simulink model "Wischer_Box17b"  (R2017b)
settings: Solver=FixedStepAuto  StartTime=0.0  StopTime=10.0  RelTol=1e-3
PreLoadFcn:
  | waijung.modelPreload; % Required for working with Waijung Blockset. Do not remove.
undefined symbols (not defined in the file): HSEOSC, Link, LQFP176, ST, STM32F417IG
libraries: simulink x12, canmsglib x6, stm32f4_canbus_lib x3, hdlsllib x2, stm32f4_io_lib x2, stm32f4_adc_lib x1, stm32f4_device_config_lib x1
CloseFcn:
  | waijung.modelClose; % Required for working with Waijung Blockset. Do not remove.
settings Model: Creator=id605605  LastModifiedBy=MichaelRogalski
settings DataIOCC: ReturnWorkspaceOutputs=on
settings OptimizationCC: DefaultParameterBehavior=Inlined  EnhancedBackFolding=on  PassReuseOutputArgsAs=Individual arguments  ZeroExternalMemoryAtStartup=off  ZeroInternalMemoryAtStartup=off  OptimizeBlockOrder=speed  DifferentSizesBufferReuse=on
settings DebuggingCC: ParameterTunabilityLossMsg=error
settings HardwareCC: ProdBitPerPointer=32  ProdBitPerSizeT=32  ProdBitPerPtrDiffT=32  ProdLargestAtomicFloat=None  ProdIntDivRoundTo=Undefined  ProdWordSize=32  ProdHWDeviceType=ARM Compatible->Cortex - M4  TargetEndianess=LittleEndian  TargetHWDeviceType=ARM Compatible->Cortex - M4
settings SFSimCC: SimUseLocalCustomCode=on  MATLABDynamicMemAlloc=off
settings RTWCC: Description=STM32F4 Target  SystemTargetFile=stm32f4.tlc  GenerateMakefile=off  TemplateMakefile=ert_default_tmf  GenerateReport=on  RTWUseLocalCustomCode=on  IncludeHyperlinkInReport=on  LaunchReport=on  GenerateTraceInfo=on  GenerateTraceReport=on  GenerateTraceReportSl=on  GenerateTraceReportSf=on  GenerateTraceReportEml=on
settings CodeAppCC: ForceParamTrailComments=on  IgnoreCustomStorageClasses=off  OperatorAnnotations=on  SimulinkDataObjDesc=on  SFDataObjDesc=on  InsertBlockDesc=on
settings STFCustomTargetCC: TargetLangStandard=C99 (ISO)  MultiwordLength=256  ModelReferenceCompliant=off  CombineOutputUpdateFcns=on  ERTCustomFileBanners=on  SupportContinuousTime=off  SupportNonInlinedSFcns=off  RemoveResetFunc=on  MATLABClassNameForMDSCustomization=Simulink.SoftwareTarget.ERTCustomization  GRTInterface=off  SystemTargetFile=stm32f4.tlc
settings ERTTargetCC: TargetLangStandard=C99 (ISO)  ModelReferenceCompliant=off  ParMdlRefBuildCompliant=off  CompOptLevelCompliant=off  ConcurrentExecutionCompliant=off  ModelStepFunctionPrototypeControlCompliant=off  CPPClassGenCompliant=off  UseToolchainInfoCompliant=off  InlinedParameterPlacement=NonHierarchical  ERTSrcFileBannerTemplate=stm32f4_code_template.cgt  ERTHdrFileBannerTemplate=stm32f4_code_template.cgt  ERTDataSrcFileTemplate=stm32f4_code_template.cgt  ERTDataHdrFileTemplate=stm32f4_code_template.cgt  ERTCustomFileTemplate=stm32f4_file_process.tlc

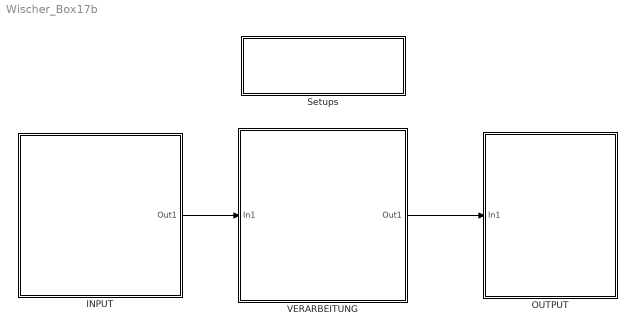
== system Wischer_Box17b ==
  INPUT : Subsystem
  OUTPUT : Subsystem
  Setups : Subsystem
  VERARBEITUNG : Subsystem
  wires:
  VERARBEITUNG/1(Out1) -> OUTPUT/1(In1)
  INPUT/1(Out1) -> VERARBEITUNG/1(In1)

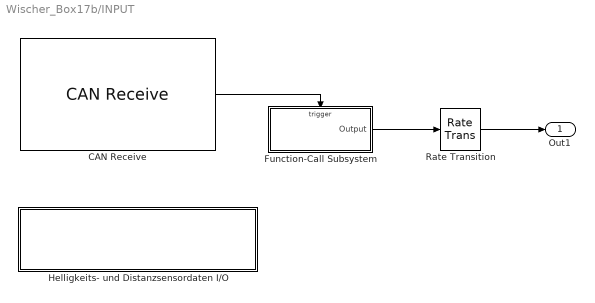
== system Wischer_Box17b/INPUT ==
  CAN Receive : stm32f4_canbus_lib/CAN Receive  conf=Rx  canmodule=1  idtype=Standard  filtertype=Mask  id=0  idmask=0  enableisr=on  usedlc=off  datatype=single  data0type=uint32  data1type=uint32  data2type=Not used  data3type=Not used  data4type=Not used  data5type=Not used  data6type=Not used  data7type=Not used  buffersize=8  sampletime=-1  sampletimestr=-1  blockid=INPUTCANReceive  inputarray=[]  inputlabelarray={}  outputarray=[7]  outputlabelarray={'Call ISR' }  compat=0  confstr=[]
      settings: SourceProductName=Waijung Blockset
  Function-Call Subsystem : Subsystem  TreatAsAtomicUnit=on
  Helligkeits- und Distanzsensordaten I/O : Subsystem
  Rate Transition : RateTransition
  Out1 : Outport  VectorParamsAs1DForOutWhenUnconnected=off
  wires:
  CAN Receive/1 -> Function-Call Subsystem/Trigger
  Function-Call Subsystem/1(Output) -> Rate Transition/1
  Rate Transition/1 -> Out1/1

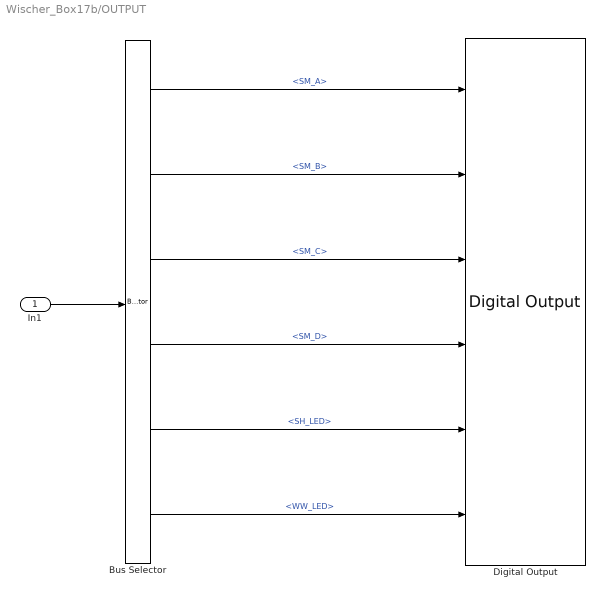
== system Wischer_Box17b/OUTPUT ==
  In1 : Inport
  Bus Selector : BusSelector  OutputSignals=SM_A,SM_B,SM_C,SM_D,SH_LED,WW_LED
  Digital Output : stm32f4_io_lib/Digital Output  use_bitband=on  port=C  speed=100  porttype=Push Pull  porttypestr=PP  use_pin0=on  use_pin1=on  use_pin2=on  use_pin3=on  use_pin4=on  use_pin5=on  use_pin6=off  use_pin7=off  use_pin8=off  use_pin9=off  use_pin10=off  use_pin11=off  use_pin12=off  use_pin13=off  use_pin14=off  use_pin15=off  pinstr=GPIO_Pin_0 | GPIO_Pin_1 | GPIO_Pin_2 | GPIO_Pin_3 | GPIO_Pin_4 | GPIO_Pin_5  usedpinarray="[1  1  1  1  1  1  0  0  0  0  0  0  0  0  0  0]"  bitbandingstr=|  sampletime=-1  sampletimestr=-1  blockid=OUTPUTDigitalOutput  enablecustomportlabel=off  globalinit=off  cinputportlabel=In1, In2  coutputportlabel=0
      | #define OUTPUTDigitalOutput_C0 Peripheral_BB(GPIOC->ODR, 0)  /* Output pin */
      | #define OUTPUTDigitalOutput_C1 Peripheral_BB(GPIOC->ODR, 1)  /* Output pin */
      | #define OUTPUTDigitalOutput_C2 Peripheral_BB(GPIOC->ODR, 2)  /* Output pin */
      | #define OUTPUTDigitalOutput_C3 Peripheral_BB(GPIOC->ODR, 3)  /* Output pin */
      | #define OUTPUTDigitalOutput_C4 Peripheral_BB(GPIOC->ODR, 4)  /* Output pin */
      | #define OUTPUTDigitalOutput_C5 Peripheral_BB(GPIOC->ODR, 5)  /* Output pin */
      settings: SourceProductName=Waijung Blockset
  wires:
  In1/1 -> Bus Selector/1
  Bus Selector/1 -> Digital Output/1  "<SM_A>"
  Bus Selector/2 -> Digital Output/2  "<SM_B>"
  Bus Selector/3 -> Digital Output/3  "<SM_C>"
  Bus Selector/4 -> Digital Output/4  "<SM_D>"
  Bus Selector/6 -> Digital Output/6  "<WW_LED>"
  Bus Selector/5 -> Digital Output/5  "<SH_LED>"

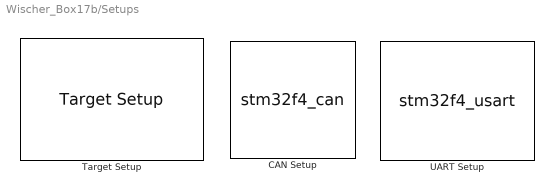
== system Wischer_Box17b/Setups ==
  CAN Setup : S-Function  FunctionName=stm32f4_can  Parameters=conf,canmodule,0,inputarray,outputarray,'','',confstr,sampletime,sampletimestr,blockid  SFunctionDeploymentMode=off  EnableBusSupport=off  mask(stm32f4_can){conf=Setup, canmodule=1, advance=off, bitrate_select=500000, sjw=1tq, bs1=14tq, bs2=6tq, timingconf=Prescaler, brp=4, bitrate=500000, tq=9.5238e-08, autoretransmission=Disable, remaptxpin=A12, remaprxpin=A11, sampletime=-1, sampletimestr=-1, blockid=SetupsCANSetup, inputarray=[], inputlabelarray={}, outputarray=[], outputlabelarray={}, compat=0, confstr=[], presc=4, txportstr=A, txpinstr=12, rxportstr=A, rxpinstr=11, lastmodule=1}
      mask prompts: conf "Configuration"; canmodule "CAN Module"; advance "Advance configuration"; bitrate_select "Baud rate (bps)"; sjw "Resync Jump Width (SJW)"; bs1 "Bit segment 1 (BS1) + PROP_SEG"; bs2 "Bit segment 2 (BS2)"; timingconf "Adjust"; brp "Baud rate prescaler (BRP)"; bitrate "Baud rate (bps)"; tq "Time Quantum (Second), tq"; autoretransmission "Auto Re-transmission"; remaptxpin "CAN Tx pin"; remaprxpin "CAN Rx pin"; sampletime "Sample time (sec)"; sampletimestr "Compiled sample time (sec) in string"; inputarray "Input port"; inputlabelarray "Input port label"; outputarray "Output port"; outputlabelarray "Output port label"; compat "Compatibility (Reserved for future use)"; confstr "Configuration String"; presc "Prescale"; txportstr "Tx port string"; txpinstr "Tx pin string"; rxportstr "Rx port string"; rxpinstr "Rx pin string"; lastmodule "Last module selected"
      mask help:
      | This block setups CAN Module.
      |
      | Auto Re-transmission,
      |  - Enable: The CAN hardware will automatically retransmit the message until it has been
      | successfully transmitted according to the CAN standard.
      |  - Disable: A message will be transmitted only once, independently of the transmission result
      | (successful, error or arbitration lost).
      mask init:
      | stm32f4_can_callback('init');
      mask Help: web(fullfile(waijungdocroot,'stm32f4_can_setup.htm'), '-browser')
      mask TypeOptions conf: Setup
      mask TypeOptions canmodule: 1 | 2
      mask Callback canmodule: stm32f4_can_callback('canmodule');
      mask Callback advance: stm32f4_can_callback('advance');
      mask TypeOptions bitrate_select: 125000 | 250000 | 500000 | 1000000
      mask Callback bitrate_select: stm32f4_can_callback('bitrate_select');
      mask TypeOptions sjw: 1tq | 2tq | 3tq | 4tq
      mask TypeOptions bs1: 1tq | 2tq | 3tq | 4tq | 5tq | 6tq | 7tq | 8tq | 9tq | 10tq | 11tq | 12tq | 13tq | 14tq | 15tq | 16tq
      mask Callback bs1: stm32f4_can_callback('timingconf');
      mask TypeOptions bs2: 1tq | 2tq | 3tq | 4tq | 5tq | 6tq | 7tq | 8tq
      mask Callback bs2: stm32f4_can_callback('timingconf');
      mask TypeOptions timingconf: Prescaler | Baudrate
      mask Callback timingconf: stm32f4_can_callback('timingconf');
      mask Callback brp: stm32f4_can_callback('timingconf');
      mask Callback bitrate: stm32f4_can_callback('timingconf');
      mask TypeOptions autoretransmission: Enable | Disable
      mask TypeOptions remaptxpin: Not used | A12 | B9 | D1 | H13
      mask Callback remaptxpin: stm32f4_can_callback('remaptxpin');
      mask TypeOptions remaprxpin: Not used | A11 | B8 | D0 | I9
      mask Callback remaprxpin: stm32f4_can_callback('remaprxpin');
      mask Callback sampletime: stm32f4_can_callback('sampletime');
      mask Callback sampletimestr: stm32f4_can_callback('sampletimestr');
      mask Callback blockid: stm32f4_can_callback('blockid');
      mask Display: text(0.5, 0.5, 'CAN1_Setup\nSpeed (bps): 500000\nTx/Rx pin: A12/A11','ver','middle','hor','center');
  Target Setup : stm32f4_device_config_lib/Target Setup  Priority=100  compiler=GNU ARM  previous_compiler=GNU ARM  mcu=STM32F417IG (LQFP176)  mcustr=STM32F417IG  clockconfig=HSEOSC-8MHz  system_stm32f4xx_c_path=D:\Downloads\waijung17_03a\targets\stm32f4_target\stm32f4\utils\system_stm32f4xx_default\STM32F40_41xxx\hseosc8mhz  showmemoryconfiguration=off  stacksize=0x2000  heapsize=0x2000  enableautocompiledownload=on  fullchiperase=off  programmerinterface=ST-Link  editctrlstr=on  compilercontrolstr=$(patsubst %, -I%, .) -mcpu=cortex-m4 -mthumb -mthumb-interwork -mfloat-abi=hard -mfpu=fpv4-sp-d16 -ffast-math -Wall -Wextra -Ofast  assemblercontrolstr=$(patsubst %, -I%, .) -mcpu=cortex-m4 -mthumb -mthumb-interwork -mfloat-abi=hard -mfpu=fpv4-sp-d16 -ffast-math -Wall -Wextra -Ofast -Wa,-amhls=$(<:.s=.lst) -D__STACK_SIZE=$(STACK_SIZE) -D__HEAP_SIZE=$(HEAP_SIZE)  linkercontrolstr=-T$(LD_SCRIPT) -g -Wl,-Map=$(MAP),--cref,--no-warn-mismatch -mcpu=cortex-m4 -mthumb -mthumb-interwork -mfloat-abi=hard -mfpu=fpv4-sp-d16 -specs=nosys.specs  runafterdownload=on  execprofile=None  profileruart=3  profilerbaud=500000  profilertxpin=D8  profilerinitstr=0.01,168000000,1680000,500000,0  manualsetsampletime=off  sampletime=0.01  blockid=SetupsTargetSetup  systickreloadvalue=1680000  hseval=8000000  lastprofileruart=3  hclk=168000000  flashorigin=0x8000000  flashlength=1024k  ramorigin=0x20000000  ramlength=128k  useextram=off
      settings: SourceProductName=Waijung Blockset
  UART Setup : S-Function  Priority=1  FunctionName=stm32f4_usart  Parameters=configuration,uartmodule,transfer,baudrate,inputtype,outputtype,confstr,binheaderarray,binterminatorarray,asciiheader,asciiterminator,bindatalength,packetmode,varname,sampletime,sampletimestr,blockid  SFunctionDeploymentMode=off  EnableBusSupport=off  mask(stm32f4_usart){configuration=Setup, uartmodule=2, baudrate=115200, databits=8, parity=No, stopbit=1, remaptxpin=A2, remaprxpin=A3, flowcontrol=None, remapctspin=Not used, remaprtspin=Not used, advanceoptions=off, rxbuffersize=512, txbuffersize=512, transfer=Blocking, packetmode=Ascii, binheader='7E 7E', binterminator='03 03', porttype_double=1, porttype_single=0, porttype_int8=1, porttype_uint8=0, porttype_int16=0, porttype_uint16=0, porttype_int32=0, porttype_uint32=0, asciiformat='%d,%f', rx_asciiterminator=CRLF (0x0D 0x0A - "\r\n"), tx_asciiterminator=CR (0x0D - "\r"), storagename=<empty>, varname=, inputtype=[0], outputtype=[0], binheaderarray=[0], binterminatorarray=[0], bindatalength=0, asciiheader='', asciiterminator=[0], sampletime=-1, sampletimestr=-1, blockid=SetupsUARTSetup, confstr=[ "dummy", "1", "A", "2", "1", "A", "3", "0", "*", "*", "0", "*", "*", "1", "4", "6", "1", "4", "5", "512", "512", "1", "2", "115200", "8", "No", "1", "None", "USART2"], lastmodule=2}
      mask prompts: uartmodule "UART Module"; baudrate "Baud rate (bps)"; databits "Data bits"; stopbit "Stop bit"; remaptxpin "Tx Pin"; remaprxpin "Rx Pin"; flowcontrol "Hardware flow control"; remapctspin "HW Flow control, CTS Pin"; remaprtspin "HW Flow control, RTS Pin"; advanceoptions "Advance options"; rxbuffersize "Rx buffer size (bytes)"; txbuffersize "Tx buffer size (bytes)"; packetmode "Packet mode"; binheader "Binary header (example: '7E 7E')"; binterminator "Binary terminator (example: '03 03')"; porttype_double "Number of data port, type DOUBLE"; porttype_single "Number of data port, type SINGLE"; porttype_int8 "Number of data port, type INT8"; porttype_uint8 "Number of data port, type UINT8"; porttype_int16 "Number of data port, type INT16"; porttype_uint16 "Number of data port, type UINT16"; porttype_int32 "Number of data port, type INT32"; porttype_uint32 "Number of data port, type UINT32"; asciiformat "Ascii format"; rx_asciiterminator "End of packet"; tx_asciiterminator "End of packet"; storagename "Buffer"; varname "Var name"; inputtype "Input data type"; outputtype "Output data type"; binheaderarray "Binary header"; binterminatorarray "Binary terminator"; bindatalength "Binary data length"; asciiheader "Ascii header (printf format)"; asciiterminator "Ascii terminator"; sampletime "Sample time (sec)"; sampletimestr "Compiled sample time (sec) in string"; confstr "Configuration string"; lastmodule "Last module selected"
      mask help:
      | Default STM32F4DISCOVERY + aMG F4 Connect 2 + aMG USB Converter N2 settings use
      |
      | USART3, Tx D8, Rx D9 and USB Serial Converter A.
      mask init:
      | stm32f4_usart_callback('init');
      mask Help: web(fullfile(waijungdocroot,'stm32f4_usart_setup.htm'), '-browser')
      mask TypeOptions configuration: Setup | Tx | Rx
      mask Callback configuration: stm32f4_usart_callback('configuration');
      mask TypeOptions uartmodule: 1 | 2 | 3 | 4 | 5 | 6
      mask Callback uartmodule: stm32f4_usart_callback('uartmodule');
      mask Callback baudrate: stm32f4_usart_callback('baudrate');
      mask TypeOptions databits: 8
      mask TypeOptions parity: No | Odd | Even
      mask TypeOptions stopbit: 0.5 | 1 | 1.5 | 2
      mask TypeOptions remaptxpin: Not used | A2 | D5
      mask TypeOptions remaprxpin: Not used | A3 | D6
      mask TypeOptions flowcontrol: None | RTS | CTS | RTS/CTS
      mask Callback flowcontrol: stm32f4_usart_callback('flowcontrol');
      mask TypeOptions remapctspin: Not used | A0 | D3
      mask TypeOptions remaprtspin: Not used | A1 | D4
      mask Callback advanceoptions: stm32f4_usart_callback('advanceoptions');
      mask TypeOptions rxbuffersize: 16 | 32 | 64 | 128 | 256 | 512 | 1024 | 2048
      mask TypeOptions txbuffersize: 16 | 32 | 64 | 128 | 256 | 512 | 1024 | 2048
      mask TypeOptions transfer: Blocking | Non-Blocking
      mask Callback transfer: stm32f4_usart_callback('transfer');
      mask TypeOptions packetmode: Ascii | Binary | String Buffer
      mask Callback packetmode: stm32f4_usart_callback('packetmode');
      mask Callback binheader: stm32f4_usart_callback('binheader');
      mask Callback binterminator: stm32f4_usart_callback('binterminator');
      mask Callback porttype_double: stm32f4_usart_callback('porttype');
      mask Callback porttype_single: stm32f4_usart_callback('porttype');
      mask Callback porttype_int8: stm32f4_usart_callback('porttype');
      mask Callback porttype_uint8: stm32f4_usart_callback('porttype');
      mask Callback porttype_int16: stm32f4_usart_callback('porttype');
      mask Callback porttype_uint16: stm32f4_usart_callback('porttype');
      mask Callback porttype_int32: stm32f4_usart_callback('porttype');
      mask Callback porttype_uint32: stm32f4_usart_callback('porttype');
      mask Callback asciiformat: stm32f4_usart_callback('asciiformat');
      mask TypeOptions rx_asciiterminator: CR (0x0D - "\r") | LF (0x0A - "\n") | CRLF (0x0D 0x0A - "\r\n")
      mask Callback rx_asciiterminator: stm32f4_usart_callback('rx_asciiterminator');
      mask TypeOptions tx_asciiterminator: CR (0x0D - "\r") | LF (0x0A - "\n") | CRLF (0x0D 0x0A - "\r\n") | None
      mask Callback tx_asciiterminator: stm32f4_usart_callback('tx_asciiterminator');
      mask TypeOptions storagename: <empty>
      mask Callback storagename: stm32f4_usart_callback('storagename');
      mask Callback varname: stm32f4_usart_callback('varname');
      mask Callback sampletime: stm32f4_usart_callback('sampletime');
      mask Callback sampletimestr: stm32f4_usart_callback('sampletimestr');
      mask Callback blockid: stm32f4_usart_callback('blockid');
      mask Display: text(0.5, 0.5, 'Module: USART2_Setup\nBaud (Bps): 115200\nDMA Buffer: 512/512\nTx/Rx Pin: A2/A3','ver','middle','hor','center');

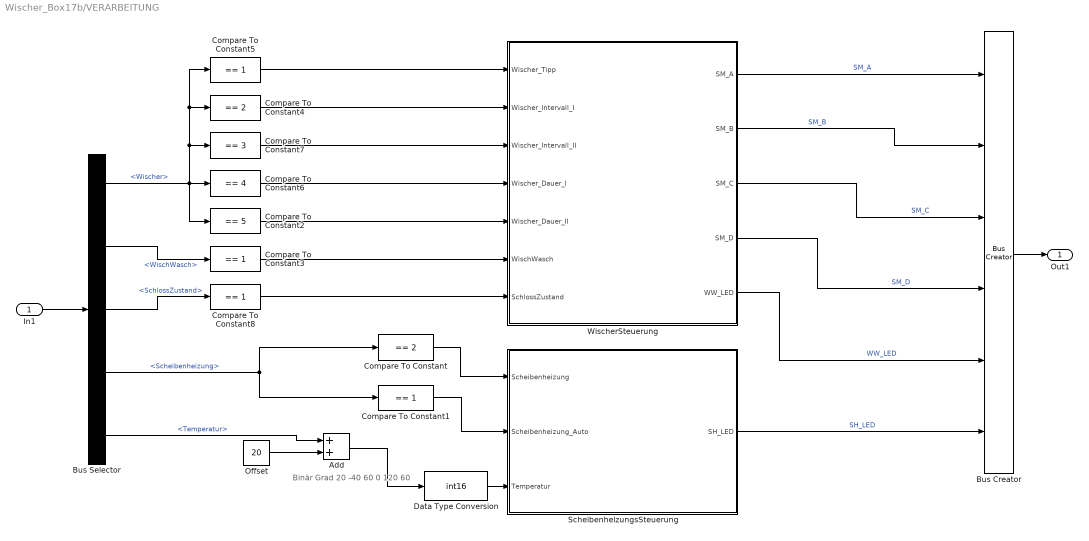
== system Wischer_Box17b/VERARBEITUNG ==
  note: Binär   Grad
      | 20		-40
      | 60		0
      | 120		60
  In1 : Inport
  Add : Sum
  Bus Creator : BusCreator  Inputs=6
  Bus Selector : BusSelector  OutputSignals=Wischer,WischWasch,SchlossZustand,Scheibenheizung,Temperatur
  Compare To Constant : simulink/Logic and Bit Operations/Compare To Constant  relop===  const=2  OutDataTypeStr=boolean
  Compare To Constant{1,3,5,8} (4 alike) : simulink/Logic and Bit Operations/Compare To Constant  relop===  const=1  OutDataTypeStr=boolean
  Compare To Constant2 : simulink/Logic and Bit Operations/Compare To Constant  relop===  const=5  OutDataTypeStr=boolean
  Compare To Constant4 : simulink/Logic and Bit Operations/Compare To Constant  relop===  const=2  OutDataTypeStr=boolean
  Compare To Constant6 : simulink/Logic and Bit Operations/Compare To Constant  relop===  const=4  OutDataTypeStr=boolean
  Compare To Constant7 : simulink/Logic and Bit Operations/Compare To Constant  relop===  const=3  OutDataTypeStr=boolean
  Data Type Conversion : DataTypeConversion  OutDataTypeStr=int16
  Offset : Constant  Value=20
  ScheibenheizungsSteuerung : Stateflow chart  TreatAsAtomicUnit=on
  WischerSteuerung : Stateflow chart  TreatAsAtomicUnit=on
  Out1 : Outport  VectorParamsAs1DForOutWhenUnconnected=off
  wires:
  Bus Creator/1 -> Out1/1
  In1/1 -> Bus Selector/1
  WischerSteuerung/1(SM_A) -> Bus Creator/1  "SM_A"
  WischerSteuerung/2(SM_B) -> Bus Creator/2  "SM_B"
  WischerSteuerung/3(SM_C) -> Bus Creator/3  "SM_C"
  WischerSteuerung/4(SM_D) -> Bus Creator/4  "SM_D"
  WischerSteuerung/5(WW_LED) -> Bus Creator/5  "WW_LED"
  ScheibenheizungsSteuerung/1(SH_LED) -> Bus Creator/6  "SH_LED"
  Bus Selector/3 -> Compare To Constant8/1  "<SchlossZustand>"
  Bus Selector/4 -> Compare To Constant/1, Compare To Constant1/1  "<Scheibenheizung>"
  Compare To Constant/1 -> ScheibenheizungsSteuerung/1(Scheibenheizung)
  Compare To Constant1/1 -> ScheibenheizungsSteuerung/2(Scheibenheizung_Auto)
  Compare To Constant7/1 -> WischerSteuerung/3(Wischer_Intervall_II)
  Compare To Constant4/1 -> WischerSteuerung/2(Wischer_Intervall_I)
  Bus Selector/1 -> Compare To Constant2/1, Compare To Constant7/1, Compare To Constant4/1, Compare To Constant5/1, Compare To Constant6/1  "<Wischer>"
  Compare To Constant6/1 -> WischerSteuerung/4(Wischer_Dauer_I)
  Compare To Constant2/1 -> WischerSteuerung/5(Wischer_Dauer_II)
  Compare To Constant5/1 -> WischerSteuerung/1(Wischer_Tipp)
  Bus Selector/2 -> Compare To Constant3/1  "<WischWasch>"
  Compare To Constant3/1 -> WischerSteuerung/6(WischWasch)
  Compare To Constant8/1 -> WischerSteuerung/7(SchlossZustand)
  Offset/1 -> Add/2
  Bus Selector/5 -> Add/1  "<Temperatur>"
  Add/1 -> Data Type Conversion/1
  Data Type Conversion/1 -> ScheibenheizungsSteuerung/3(Temperatur)

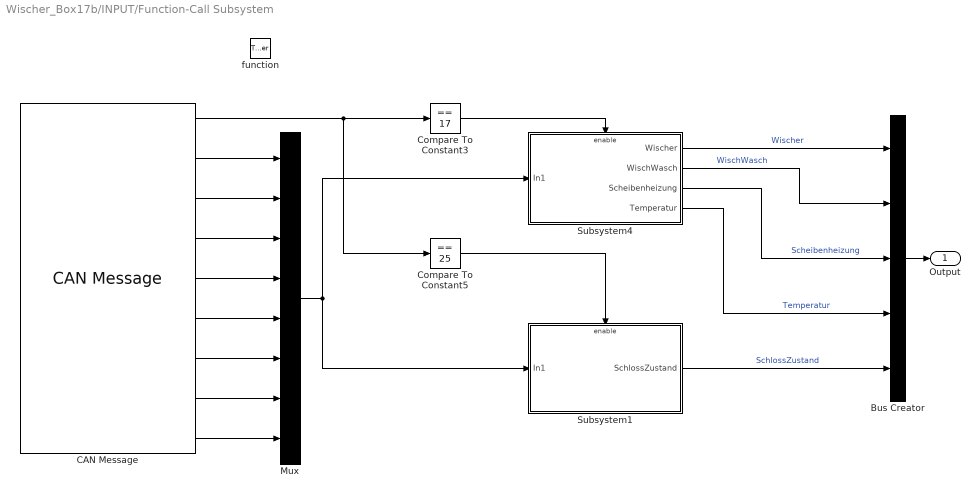
== system Wischer_Box17b/INPUT/Function-Call Subsystem ==
  function : TriggerPort  TriggerType=function-call  VariantControl=Variant
  Bus Creator : BusCreator  Inputs=5
  CAN Message : stm32f4_canbus_lib/CAN Message  conf=Msg  canmodule=1  usedlc=off  datatype=double  data0type=uint8  data1type=uint8  data2type=uint8  data3type=uint8  data4type=uint8  data5type=uint8  data6type=uint8  data7type=uint8  sampletime=-1  sampletimestr=-1  blockid=INPUTFunctionCallSubsystemCANMessage  inputarray=[]  inputlabelarray={}  outputarray=[ 7, 3, 3, 3, 3, 3, 3, 3, 3]  outputlabelarray={'ID', 'D0 (uint8)', 'D1 (uint8)', 'D2 (uint8)', 'D3 (uint8)', 'D4 (uint8)', 'D5 (uint8)', 'D6 (uint8)', 'D7 (uint8)' }  compat=0  confstr=[]
      settings: SourceProductName=Waijung Blockset
  Compare To Constant3 : simulink/Logic and Bit Operations/Compare To Constant  relop===  const=17  OutDataTypeStr=boolean
  Compare To Constant5 : simulink/Logic and Bit Operations/Compare To Constant  relop===  const=25  OutDataTypeStr=boolean
  Mux : Mux  Inputs=8
  Subsystem1 : Subsystem
  Subsystem4 : Subsystem
  Output : Outport  VectorParamsAs1DForOutWhenUnconnected=off
  wires:
  CAN Message/1 -> Compare To Constant5/1, Compare To Constant3/1
  CAN Message/3 -> Mux/2
  CAN Message/2 -> Mux/1
  CAN Message/4 -> Mux/3
  CAN Message/5 -> Mux/4
  CAN Message/6 -> Mux/5
  CAN Message/7 -> Mux/6
  CAN Message/8 -> Mux/7
  CAN Message/9 -> Mux/8
  Bus Creator/1 -> Output/1
  Compare To Constant3/1 -> Subsystem4/Enable
  Mux/1 -> Subsystem4/1(In1), Subsystem1/1(In1)
  Compare To Constant5/1 -> Subsystem1/Enable
  Subsystem4/1(Wischer) -> Bus Creator/1  "Wischer"
  Subsystem4/2(WischWasch) -> Bus Creator/2  "WischWasch"
  Subsystem4/3(Scheibenheizung) -> Bus Creator/3  "Scheibenheizung"
  Subsystem4/4(Temperatur) -> Bus Creator/4  "Temperatur"
  Subsystem1/1(SchlossZustand) -> Bus Creator/5  "SchlossZustand"

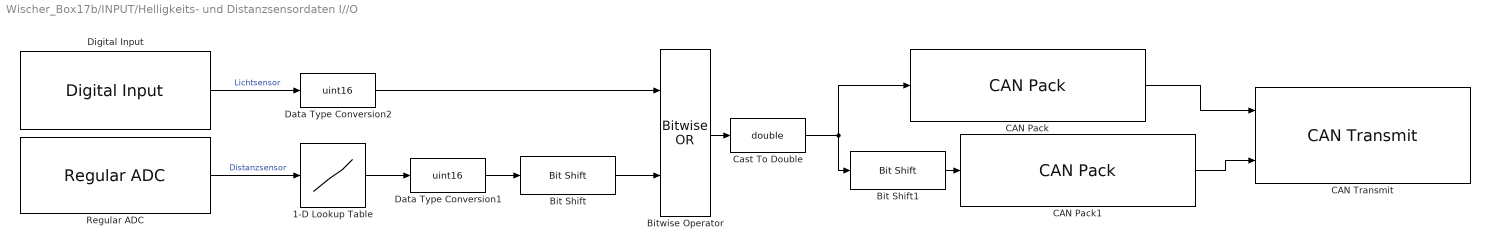
== system Wischer_Box17b/INPUT/Helligkeits- und Distanzsensordaten I//O ==
  1-D Lookup Table : Lookup_n-D  NumberOfTableDimensions=1  BreakpointsForDimension1=[310,3800]  IndexSearchMethod=Linear search  Table=[500,0]  InternalRulePriority=Speed  RndMeth=Simplest  InputSameDT=on
  Bit Shift : hdlsllib/Logic and Bit Operations/Bit Shift  mode=Shift Left Logical  N=1
      settings: SourceProductName=Simulink
  Bit Shift1 : hdlsllib/Logic and Bit Operations/Bit Shift  mode=Shift Right Logical  N=8
      settings: SourceProductName=Simulink
  Bitwise Operator : simulink/Logic and Bit Operations/Bitwise Operator  logicop=OR  UseBitMask=off  NumInputPorts=2  BitMask=bin2dec('11011001')  BitMaskRealWorld=Stored Integer
  CAN Pack : canmsglib/CAN Pack  MsgList=(none)  MsgName=CAN_Data_Sensor1  MsgIDType=Standard (11-bit identifier)  MsgIdentifier=32  MsgLength=1  Remote=off  ApplyMinMax=off  BusOutput=off  NSignals=0  StartBits=0  SignalSizes=0  ByteOrders=0  DataTypes=0  MultiplexTypes=0  MultiplexValues=0  Factors=0  Offsets=0  Minimums=0  Maximums=0
      settings: SourceProductName=Simulink Real-Time  SourceProductBaseCode=XP  DataFormat=raw data
  CAN Pack1 : canmsglib/CAN Pack  MsgList=(none)  MsgName=CAN_Data_Sensor1  MsgIDType=Standard (11-bit identifier)  MsgIdentifier=32  MsgLength=1  Remote=off  ApplyMinMax=off  BusOutput=off  NSignals=0  StartBits=0  SignalSizes=0  ByteOrders=0  DataTypes=0  MultiplexTypes=0  MultiplexValues=0  Factors=0  Offsets=0  Minimums=0  Maximums=0
      settings: SourceProductName=Simulink Real-Time  SourceProductBaseCode=XP  DataFormat=raw data
  CAN Transmit : stm32f4_canbus_lib/CAN Transmit  conf=Tx  canmodule=1  transfer=Blocking  timeout=0.005  idtype=Standard  specificid=on  id=32  specificdlc=on  dlc=2  enablestatus=off  datatype=single  data0type=uint8  data1type=uint8  data2type=Not used  data3type=Not used  data4type=Not used  data5type=Not used  data6type=Not used  data7type=Not used  inputarray=[ 3, 3]  inputlabelarray={ 'D0 (uint8)', 'D1 (uint8)' }  outputarray=[]  outputlabelarray={}  sampletime=-1  sampletimestr=-1  blockid=INPUTHelligkeitsundDistanzsensordatenIOCANTransmit  compat=0  confstr=[]
      settings: SourceProductName=Waijung Blockset
  Cast To Double : DataTypeConversion  OutDataTypeStr=double
  Data Type Conversion1 : DataTypeConversion  OutDataTypeStr=uint16
  Data Type Conversion2 : DataTypeConversion  OutDataTypeStr=uint16
  Digital Input : stm32f4_io_lib/Digital Input  port=C  speed=100  porttype=None  porttypestr=NOPULL  use_pin0=off  use_pin1=off  use_pin2=off  use_pin3=off  use_pin4=off  use_pin5=off  use_pin6=on  use_pin7=off  use_pin8=off  use_pin9=off  use_pin10=off  use_pin11=off  use_pin12=off  use_pin13=off  use_pin14=off  use_pin15=off  pinstr=GPIO_Pin_6  usedpinarray="[0  0  0  0  0  0  1  0  0  0  0  0  0  0  0  0]"  bitbandingstr="#define INPUTHelligkeitsundDistanzsensordatenIODigitalInput_C6 Peripheral_BB(GPIOC->IDR, 6)  /* Output pin */"  sampletime=-1  sampletimestr=-1  blockid=INPUTHelligkeitsundDistanzsensordatenIODigitalInput  enablecustomportlabel=off  glabalinit=off  cinputportlabel=In1, In2  coutputportlabel=Out1, Out2
      settings: SourceProductName=Waijung Blockset
  Regular ADC : stm32f4_adc_lib/Regular ADC  adcmodule=1  outputdatatype=Double  prescaler=Auto  prescalerstr=ADC_Prescaler_Div6  chsamplingtime=Auto  chsamplingtimestr=ADC_SampleTime_480Cycles  read_an0=on  read_an1=off  read_an2=off  read_an3=off  read_an4=off  read_an5=off  read_an6=off  read_an7=off  read_an8=off  read_an9=off  read_an10=off  read_an11=off  read_an12=off  read_an13=off  read_an14=off  read_an15=off  read_an16=off  read_an17=off  read_an18=off  pinstr=GPIO_Pin_0  usedpinarray="[1  0  0  0  0  0  0  0  0  0  0  0  0  0  0  0  0  0  0]"  usedportidarray=[0]  usedpinidarray=[0]  usedpinidcount=1  sampletime=-1  blockid=INPUTHelligkeitsundDistanzsensordatenIORegularADC  enablecustomportlabel=off  cinputportlabel=0  coutputportlabel=Out1, Out2
      settings: SourceProductName=Waijung Blockset
  wires:
  Cast To Double/1 -> Bit Shift1/1, CAN Pack/1
  1-D Lookup Table/1 -> Data Type Conversion1/1
  Bitwise Operator/1 -> Cast To Double/1
  Bit Shift/1 -> Bitwise Operator/2
  Data Type Conversion2/1 -> Bitwise Operator/1
  Data Type Conversion1/1 -> Bit Shift/1
  Regular ADC/1 -> 1-D Lookup Table/1  "Distanzsensor"
  Digital Input/1 -> Data Type Conversion2/1  "Lichtsensor"
  CAN Pack/1 -> CAN Transmit/1
  CAN Pack1/1 -> CAN Transmit/2
  Bit Shift1/1 -> CAN Pack1/1

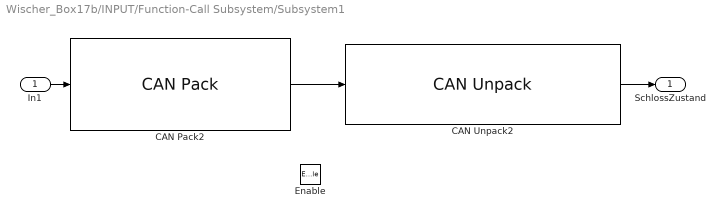
== system Wischer_Box17b/INPUT/Function-Call Subsystem/Subsystem1 ==
  In1 : Inport
  Enable : EnablePort
  CAN Pack2 : canmsglib/CAN Pack  MsgList=(none)  MsgName=CAN_Data_Schloss1  MsgIDType=Standard (11-bit identifier)  MsgIdentifier=25  MsgLength=1  Remote=off  ApplyMinMax=off  BusOutput=off  NSignals=0  StartBits=0  SignalSizes=0  ByteOrders=0  DataTypes=0  MultiplexTypes=0  MultiplexValues=0  Factors=0  Offsets=0  Minimums=0  Maximums=0
      settings: SourceProductName=Simulink Real-Time  SourceProductBaseCode=XP  DataFormat=raw data
  CAN Unpack2 : canmsglib/CAN Unpack  MsgList=(none)  MsgName=CAN_Data_Schloss1  MsgIDType=Standard (11-bit identifier)  MsgIdentifier=25  MsgLength=1  SignalInfo=SchlossZustand$0$1$1$2$1$0$1$0$-Inf$Inf$#  IDPort=off  TimestampPort=off  ErrorPort=off  RemotePort=off  LengthPort=off  StatusPort=off  ApplyMinMax=off  NSignals=1  StartBits=str2num('[int32(0)]')  SignalSizes=str2num('[int32(1)]')  ByteOrders=str2num('[int32(1)]')  DataTypes=str2num('[int32(2)]')  MultiplexTypes=str2num('[int32(1)]')  MultiplexValues=str2num('[double(0)]')  Factors=str2num('[double(1)]')  Offsets=str2num('[double(0)]')  Minimums=str2num('[double(-Inf)]')  Maximums=str2num('[double(Inf)]')
      settings: SourceProductName=Simulink Real-Time  SourceProductBaseCode=XP
  SchlossZustand : Outport  VectorParamsAs1DForOutWhenUnconnected=off
  wires:
  CAN Pack2/1 -> CAN Unpack2/1
  In1/1 -> CAN Pack2/1
  CAN Unpack2/1 -> SchlossZustand/1

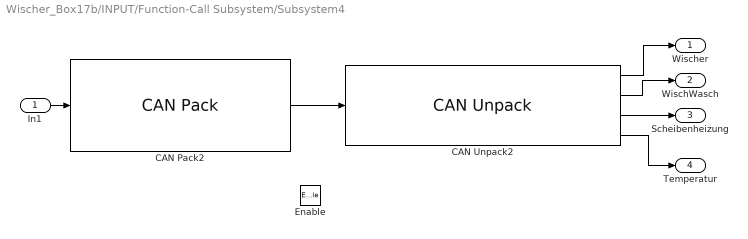
== system Wischer_Box17b/INPUT/Function-Call Subsystem/Subsystem4 ==
  In1 : Inport
  Enable : EnablePort
  CAN Pack2 : canmsglib/CAN Pack  MsgList=(none)  MsgName=CAN_Data_Cockpit2  MsgIDType=Standard (11-bit identifier)  MsgIdentifier=17  MsgLength=1  Remote=off  ApplyMinMax=off  BusOutput=off  NSignals=0  StartBits=0  SignalSizes=0  ByteOrders=0  DataTypes=0  MultiplexTypes=0  MultiplexValues=0  Factors=0  Offsets=0  Minimums=0  Maximums=0
      settings: SourceProductName=Simulink Real-Time  SourceProductBaseCode=XP  DataFormat=raw data
  CAN Unpack2 : canmsglib/CAN Unpack  MsgList=(none)  MsgName=CAN_Data_Cockpit2  MsgIDType=Standard (11-bit identifier)  MsgIdentifier=17  MsgLength=2  SignalInfo=Wischer$0$3$1$2$1$0$1$0$-Inf$Inf$#WischWasch$3$1$1$2$1$0$1$0$-Inf$Inf$#Scheibenheizung$4$2$1$2$1$0$1$0$-Inf$Inf$#Temperatur$6$7$1$2$1$0$1$0$-Inf$Inf$#  IDPort=off  TimestampPort=off  ErrorPort=off  RemotePort=off  LengthPort=off  StatusPort=off  ApplyMinMax=off  NSignals=4  StartBits=str2num('[int32(0);int32(3);int32(4);int32(6)]')  SignalSizes=str2num('[int32(3);int32(1);int32(2);int32(7)]')  ByteOrders=str2num('[int32(1);int32(1);int32(1);int32(1)]')  DataTypes=str2num('[int32(2);int32(2);int32(2);int32(2)]')  MultiplexTypes=str2num('[int32(1);int32(1);int32(1);int32(1)]')  MultiplexValues=str2num('[double(0);double(0);double(0);double(0)]')  Factors=str2num('[double(1);double(1);double(1);double(1)]')  Offsets=str2num('[double(0);double(0);double(0);double(0)]')  Minimums=str2num('[double(-Inf);double(-Inf);double(-Inf);double(-Inf)]')  Maximums=str2num('[double(Inf);double(Inf);double(Inf);double(Inf)]')
      settings: SourceProductName=Simulink Real-Time  SourceProductBaseCode=XP
  Wischer : Outport  VectorParamsAs1DForOutWhenUnconnected=off
  WischWasch : Outport  Port=2  VectorParamsAs1DForOutWhenUnconnected=off
  Scheibenheizung : Outport  Port=3  VectorParamsAs1DForOutWhenUnconnected=off
  Temperatur : Outport  Port=4  VectorParamsAs1DForOutWhenUnconnected=off
  wires:
  In1/1 -> CAN Pack2/1
  CAN Pack2/1 -> CAN Unpack2/1
  CAN Unpack2/1 -> Wischer/1
  CAN Unpack2/2 -> WischWasch/1
  CAN Unpack2/3 -> Scheibenheizung/1
  CAN Unpack2/4 -> Temperatur/1

== stateflow chart Wischer_Box17b/VERARBEITUNG/WischerSteuerung ==
  state Wischer
    en, du: wisher_cnt = 0
    state Dauer_Schnell
      en, du: wischen = true
      frequency = 0.01852
      wisher_delay = 0
    state Dauer_Langsam
      en, du: wischen = true
      frequency = 0.03704
      wisher_delay = 0
    state OFF
      en, du: wischen = false
      wisher_delay = 0
    state Intervall_Langsam
      en, du: wischen = true
      frequency = 0.03704
      wisher_delay = 4
    state Intervall_Schnell
      en, du: wischen = true
      frequency = 0.03704
      wisher_delay = 2
    state Tipp
      en, du: wischen = true
      frequency = 0.03704
      wisher_delay = 0
    state Wisch_Wasch_Aktivierung
      en, du:
      if SchlossZustand == true
      WischWaschActive = true
      end
      Interrupt = false
      frequency = 0.03704
      wisher_delay = 0
      wisher_cnt = 3
    (junction 402) -> Dauer_Schnell [order 3] : [Wischer_Dauer_II]
    (junction 402) -> Dauer_Langsam [order 2] : [Wischer_Dauer_I]
    (default) -> (junction 402)
    (junction 402) -> OFF [order 7]
    Wischer -> (junction 402) [order 1]
    (junction 402) -> Intervall_Langsam [order 5] : [Wischer_Intervall_I]
    (junction 402) -> Intervall_Schnell [order 4] : [Wischer_Intervall_II]
    (junction 402) -> Tipp [order 6] : [Wischer_Tipp]
    (junction 402) -> Wisch_Wasch_Aktivierung [order 1] : [WischWasch || Interrupt]
  state State_MotorWischen1
    en, du: if counter==27
    linkslauf = true
    end
    if WischWasch == true
    Interrupt = true
    end
    state Dummy
      entry:
      SM_A=true;
      SM_B=true;
      SM_C=false;
      SM_D=false;
    state Dummy1
      entry:
      SM_A=false;
      SM_B=true;
      SM_C=true;
      SM_D=false;
    state Dummy3
      entry:
      SM_A=true;
      SM_B=false;
      SM_C=false;
      SM_D=true;
    state Dummy2
      entry:
      SM_A=false;
      SM_B=false;
      SM_C=true;
      SM_D=true;
    (default) -> Dummy
    Dummy -> Dummy1 [order 1] : [linkslauf == 0 && counter <= 27 && after(frequency,sec)]{counter = counter + 1}
    Dummy1 -> Dummy [order 2] : [linkslauf == 1 && counter <= 54 && after(frequency,sec)]{counter = counter + 1}
    Dummy3 -> Dummy [order 1] : [linkslauf == 0 && counter <= 27 && after(frequency,sec)]{counter = counter + 1}
    Dummy -> Dummy3 [order 2] : [linkslauf == 1 && counter <= 54 && after(frequency,sec)]{counter = counter + 1}
    Dummy2 -> Dummy1 [order 2] : [linkslauf == 1 && counter <= 54 && after(frequency,sec)]{counter = counter + 1}
    Dummy1 -> Dummy2 [order 1] : [linkslauf == 0 && counter <= 27 && after(frequency,sec)]{counter = counter + 1}
    Dummy3 -> Dummy2 [order 2] : [linkslauf == 1 && counter <= 54 && after(frequency,sec)]{counter = counter + 1}
    Dummy2 -> Dummy3 [order 1] : [linkslauf == 0 && counter <= 27 && after(frequency,sec)]{counter = counter + 1}
  note: 1s Wischen:
      | frequency = 0.01852
  note: 2s Wischen:
      | frequency = 0.03704
  state State_Delay
  state Wisch_Wasch_LED
    en, du: WW_LED = true
  state Wisch_Wasch
    en, du:
    WW_LED = false
  (default) -> Wischer : {WischWaschActive = false, Interrupt = false}
  Wischer -> State_MotorWischen1 [order 2] : [wischen == true]{counter = 0, linkslauf = false}
  State_MotorWischen1 -> State_Delay : [counter == 55]{wischen = false}
  Wisch_Wasch -> State_MotorWischen1 [order 1] : [wisher_cnt > 0]{counter = 0, linkslauf = false}
  State_Delay -> Wischer [order 2] : after(wisher_delay, sec)
  State_Delay -> Wisch_Wasch [order 1] : [WischWaschActive == true]{wisher_cnt = wisher_cnt - 1}
  Wisch_Wasch -> Wischer [order 2] : [wisher_cnt == 0]{WischWaschActive = false}
  Wischer -> Wisch_Wasch_LED [order 1] : [WischWaschActive == true]
  Wisch_Wasch_LED -> Wisch_Wasch : [after(2,sec)]
  data: Wischer_Tipp input; Wischer_Intervall_I input; Wischer_Intervall_II input; Wischer_Dauer_I input; Wischer_Dauer_II input; WischWasch input; SM_A output; SM_B output; SM_C output; SM_D output; WW_LED output; Steps local; Forward local; StepTime local; StepTime1 local; wisher_delay local double; wisher_cnt local uint8; wisher_dir local boolean; wisher_active local boolean; wisher_timeout local double; frequency local double; counter local double; linkslauf local boolean; Pause local double; wischen local boolean; WischWaschActive local boolean; Interrupt local boolean; SchlossZustand input uint16

== stateflow chart Wischer_Box17b/VERARBEITUNG/ScheibenheizungsSteuerung ==
  state State_WaitForDeactivateButton
    entry: SH_LED=false
  state State_OFF
    entry:
    SH_LED=false
  state State_Auto
    entry: SH_LED=true
  state State_Manuell
    entry:
    SH_LED=true
  State_Manuell -> State_WaitForDeactivateButton [order 1] : [after(30,sec)]
  State_WaitForDeactivateButton -> State_OFF : [Scheibenheizung == false]
  (default) -> State_OFF
  State_OFF -> State_Auto [order 2] : [Scheibenheizung_Auto == true && Temperatur < 62]
  State_Manuell -> State_OFF [order 2] : [Scheibenheizung == false]
  State_OFF -> State_Manuell [order 1] : [Scheibenheizung == true]
  State_Auto -> State_OFF : [Scheibenheizung_Auto == false || after(30,sec)]
  data: Scheibenheizung input; Scheibenheizung_Auto input; Temperatur input; SH_LED output
